simulink model "ModeleEPOSslx"  (R2023a)
settings: Solver=VariableStepAuto  StartTime=0.0  StopTime=10.0  RelTol=1e-3
values from neighbouring files (symbols this model uses):
  J = 0.00001    (= 1e-05)    [parametres.m]
  K = 0.001    [parametres.m]
  KD_SI = 80e-6 * KD_Position    (= 0)    [parametres.m]
  KI_Courant = 0    [parametres.m]
  KI_Position = 0    [parametres.m]
  KI_Vitesse = 0    [parametres.m]
  KP_Courant = 0    [parametres.m]
  KP_Position = 0    [parametres.m]
  KP_SI = 10e-3 * KP_Position    (= 0)    [parametres.m]
  KP_Vitesse = 0    [parametres.m]
  L = 1e-3    (= 0.001)    [parametres.m]
  R = 1    [parametres.m]
settings Model: Creator=xavier.pessoles2  LastModifiedBy=xavier.pessoles2

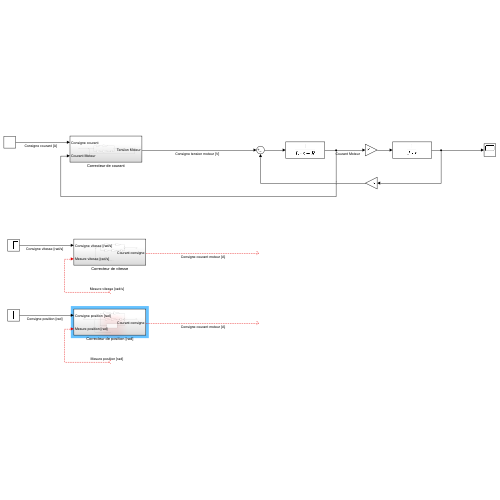
[thumbnail: Simulink's stored preview of the top-level diagram]
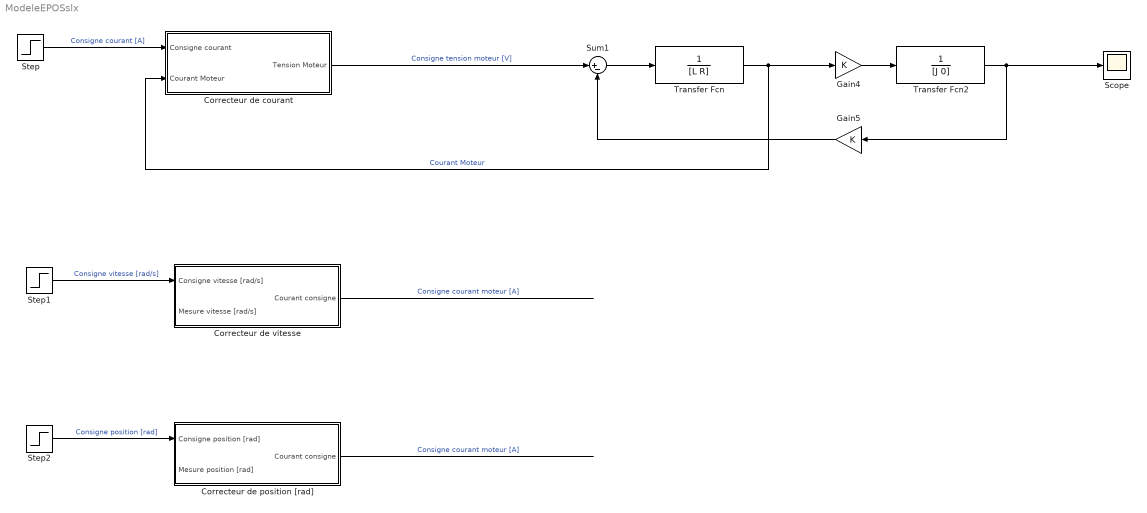
== system ModeleEPOSslx ==
  Correcteur de courant : Subsystem
  Correcteur de position [rad] : Subsystem
  Correcteur de vitesse : Subsystem
  Gain4 : Gain  Gain=K
  Gain5 : Gain  Gain=K
  Scope : Scope
  Step : Step  Time=0  SampleTime=0
  Step1 : Step  Time=0  SampleTime=0
  Step2 : Step  Time=0  SampleTime=0
  Sum1 : Sum  Inputs=|+-
  Transfer Fcn : TransferFcn  Denominator=[L R]
  Transfer Fcn2 : TransferFcn  Denominator=[J 0]
  wires:
  Sum1/1 -> Transfer Fcn/1
  Transfer Fcn/1 -> Correcteur de courant/2(Courant Moteur), Gain4/1  "Courant Moteur"
  Gain4/1 -> Transfer Fcn2/1
  Transfer Fcn2/1 -> Scope/1, Gain5/1
  Gain5/1 -> Sum1/2
  Step/1 -> Correcteur de courant/1(Consigne courant)  "Consigne courant [A]"
  Correcteur de courant/1(Tension Moteur) -> Sum1/1  "Consigne tension moteur [V]"
  Correcteur de vitesse/1(Courant consigne) -> ?  "Consigne courant moteur [A]"
  Step1/1 -> Correcteur de vitesse/1(Consigne vitesse [rad/s])  "Consigne vitesse [rad/s]"
  ? -> Correcteur de vitesse/2(Mesure vitesse [rad/s])  "Mesure vitesse [rad/s]"
  ? -> Correcteur de position [rad]/2(Mesure position [rad])  "Mesure position [rad]"
  Step2/1 -> Correcteur de position [rad]/1(Consigne position [rad])  "Consigne position [rad]"
  Correcteur de position [rad]/1(Courant consigne) -> ?  "Consigne courant moteur [A]"

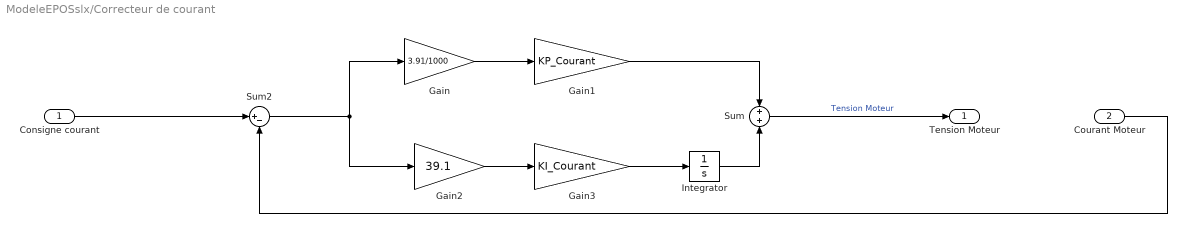
== system ModeleEPOSslx/Correcteur de courant ==
  Consigne courant : Inport
  Courant Moteur : Inport  Port=2
  Gain : Gain  Gain=3.91/1000
  Gain1 : Gain  Gain=KP_Courant
  Gain2 : Gain  Gain=39.1
  Gain3 : Gain  Gain=KI_Courant
  Integrator : Integrator
  Sum : Sum  Inputs=+|+
  Sum2 : Sum  Inputs=|+-
  Tension Moteur : Outport
  wires:
  Sum2/1 -> Gain2/1, Gain/1
  Gain3/1 -> Integrator/1
  Consigne courant/1 -> Sum2/1
  Gain2/1 -> Gain3/1
  Integrator/1 -> Sum/2
  Gain/1 -> Gain1/1
  Gain1/1 -> Sum/1
  Sum/1 -> Tension Moteur/1  "Tension Moteur"
  Courant Moteur/1 -> Sum2/2

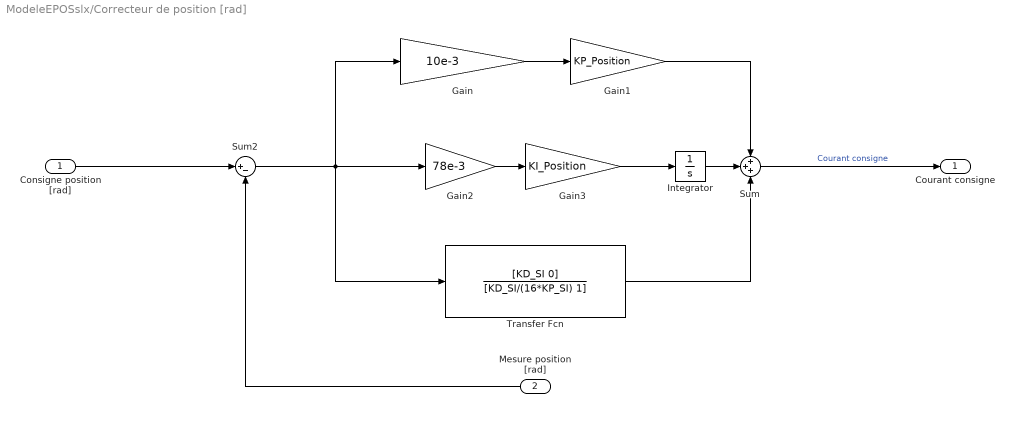
== system ModeleEPOSslx/Correcteur de position [rad] ==
  Consigne position [rad] : Inport
  Mesure position [rad] : Inport  Port=2
  Gain : Gain  Gain=10e-3
  Gain1 : Gain  Gain=KP_Position
  Gain2 : Gain  Gain=78e-3
  Gain3 : Gain  Gain=KI_Position
  Integrator : Integrator
  Sum : Sum  Inputs=+++
  Sum2 : Sum  Inputs=|+-
  Transfer Fcn : TransferFcn  Numerator=[KD_SI 0]  Denominator=[KD_SI/(16*KP_SI) 1]
  Courant consigne : Outport
  wires:
  Sum2/1 -> Gain/1, Transfer Fcn/1, Gain2/1
  Gain3/1 -> Integrator/1
  Consigne position [rad]/1 -> Sum2/1
  Gain2/1 -> Gain3/1
  Integrator/1 -> Sum/2
  Gain/1 -> Gain1/1
  Gain1/1 -> Sum/1
  Sum/1 -> Courant consigne/1  "Courant consigne"
  Mesure position [rad]/1 -> Sum2/2
  Transfer Fcn/1 -> Sum/3

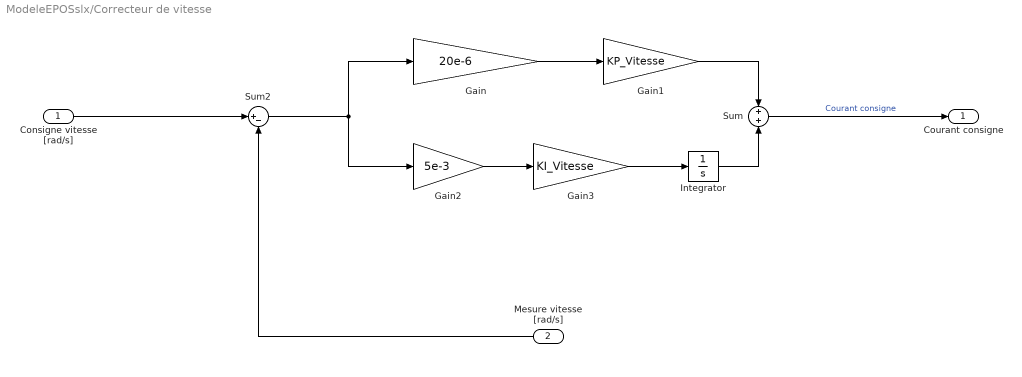
== system ModeleEPOSslx/Correcteur de vitesse ==
  Consigne vitesse [rad/s] : Inport
  Mesure vitesse [rad/s] : Inport  Port=2
  Gain : Gain  Gain=20e-6
  Gain1 : Gain  Gain=KP_Vitesse
  Gain2 : Gain  Gain=5e-3
  Gain3 : Gain  Gain=KI_Vitesse
  Integrator : Integrator
  Sum : Sum  Inputs=+|+
  Sum2 : Sum  Inputs=|+-
  Courant consigne : Outport
  wires:
  Mesure vitesse [rad/s]/1 -> Sum2/2
  Sum/1 -> Courant consigne/1  "Courant consigne"
  Gain1/1 -> Sum/1
  Gain/1 -> Gain1/1
  Integrator/1 -> Sum/2
  Gain2/1 -> Gain3/1
  Consigne vitesse [rad/s]/1 -> Sum2/1
  Gain3/1 -> Integrator/1
  Sum2/1 -> Gain/1, Gain2/1
